simulink subsystem "yarn_winding_virtual_sensor"  (R2023b)
settings: Solver=VariableStepAuto  StartTime=0.0  StopTime=10.0  RelTol=1e-3
values from neighbouring files (symbols this model uses):
  tau_s = 0.0005    [mdl_parameters_int.mat]
settings Model: Creator=Previ  LastModifiedBy=Previ

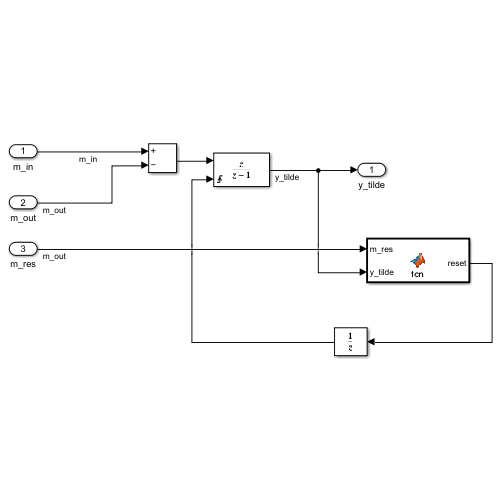
[thumbnail: Simulink's stored preview of the top-level diagram]
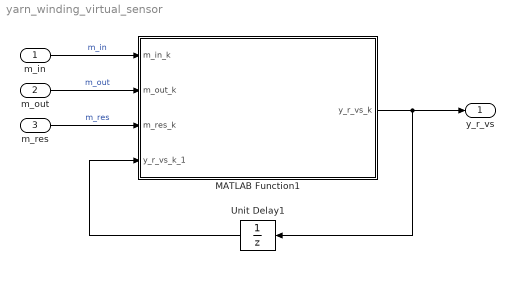
== system yarn_winding_virtual_sensor ==
  m_in : Inport  PortDimensions=[1, 1]
  m_out : Inport  Port=2  PortDimensions=[1, 1]
  m_res : Inport  Port=3  PortDimensions=[1, 1]
  MATLAB Function1 : MATLAB Function  TreatAsAtomicUnit=on
  Unit Delay1 : UnitDelay  SampleTime=tau_s  HasFrameUpgradeWarning=on
  y_r_vs : Outport  PortDimensions=[1, 1]
  wires:
  MATLAB Function1/1(y_r_vs_k) -> Unit Delay1/1, y_r_vs/1
  m_in/1 -> MATLAB Function1/1(m_in_k)  "m_in"
  m_out/1 -> MATLAB Function1/2(m_out_k)  "m_out"
  m_res/1 -> MATLAB Function1/3(m_res_k)  "m_res"
  Unit Delay1/1 -> MATLAB Function1/4(y_r_vs_k_1)

== matlab function yarn_winding_virtual_sensor/MATLAB Function1 ==
  data: m_in_k input; y_r_vs_k output; m_out_k input; m_res_k input; y_r_vs_k_1 input
function y_r_vs_k = yarnWindingVirtualSensor(m_in_k, m_out_k, m_res_k, y_r_vs_k_1)
% Update number of windings
y_r_vs_tilde_k = y_r_vs_k_1 + m_in_k - m_out_k;
if m_res_k == 1 && y_r_vs_tilde_k < 0
    % The final yarn winding is below IR2 or further
    % but the virtual sensor is in disagreement
    y_r_vs_k = 0;
elseif m_res_k == 0 && y_r_vs_tilde_k > 0
    % The final yarn winding is before IR2
    % but the virtual sensor is in disagreement
    y_r_vs_k = 0;
else
    % Do nothing
    y_r_vs_k = y_r_vs_tilde_k;
end
end
